simulink model "testLog"  (R2025a)
settings: Solver=FixedStepAuto  StartTime=0.0  StopTime=10.0  RelTol=1e-3
settings Model: Creator=grouleau  LastModifiedBy=grouleau

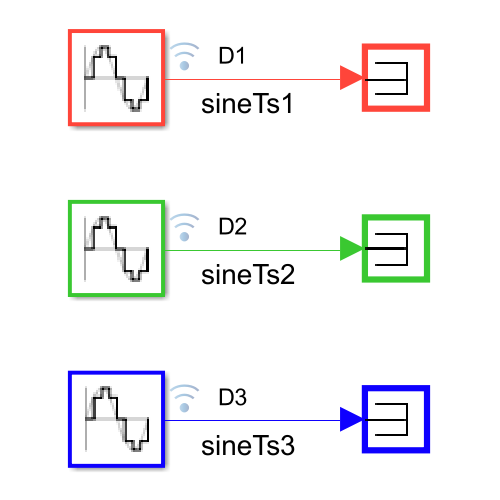
[thumbnail: Simulink's stored preview of the top-level diagram]
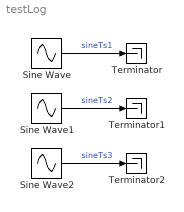
== system testLog ==
  Sine Wave : Sin  Frequency=2*pi*0.01  SampleTime=1
  Sine Wave1 : Sin  Frequency=2*pi*0.01  SampleTime=2
  Sine Wave2 : Sin  Frequency=2*pi*0.01  SampleTime=3
  Terminator : Terminator
  Terminator1 : Terminator
  Terminator2 : Terminator
  wires:
  Sine Wave/1 -> Terminator/1  "sineTs1"
  Sine Wave1/1 -> Terminator1/1  "sineTs2"
  Sine Wave2/1 -> Terminator2/1  "sineTs3"
